simulink model "OMPC"  (R2022b)
settings: Solver=ode5  StartTime=0.0  StopTime=50  FixedStep=Ts  RelTol=1e-3
values from neighbouring files (symbols this model uses):
  A = [A zeros(nA, nAm); zeros(nAm, nA) Am]    [generateFloor.m]    (also in model_floorConjuction.m = A0; model_levelConjuction.m = A0; ompc_data.m = [-0.9146 0 0.0405)
  B = [B zeros(nA, nBm); zeros(nAm, nB) Bm]    [generateFloor.m]    (also in model_floorConjuction.m = B0; model_levelConjuction.m = B0; ompc_data.m = [0.0544 -0.0757)
  Bd = Bd(:, 1:size(B, 2))    [plik_generujDane.m]
  C = [C zeros(nC, nAm); zeros(nCm, nA) Cm]    [generateFloor.m]    (also in model_floorConjuction.m = C0; model_levelConjuction.m = C0; ompc_data.m = [0.3 0.01 -0.05)
  D = Dm    [generateFloor.m]    (also in ompc_data.m = zeros(size(C,1),size(B,2)))
  G = G'    [ompc_data.m]
  nc = 4    [ompc_data.m]    (also in plik_generujDane.m = 60)
  npred = 20    [ompc_data.m]    (also in plik_generujDane.m = 120)
  nu = size(B,2)    [ompc_cost.m]    (also in ompc_cost_tracking.m; ompc_data.m; ompc_law.m; ompc_law_tracking.m)
  nx = size(B,1)    [ompc_cost.m]    (also in ompc_cost_tracking.m = size(A,1); ompc_data.m = size(A,1); ompc_law.m = size(A,1); ompc_law_tracking.m = size(A,1))
  Sc = Spsi(nx+1:end,nx+1:end)    [ompc_cost.m]    (also in ompc_cost_tracking.m = Spsi(nx+1:nx+nuc,nx+1:nx+nuc); ompc_law.m = (Sc+Sc')/2; ompc_law_tracking.m = (Sc+Sc')/2)
  Sx = Spsi(1:nx,1:nx)    [ompc_cost.m]    (also in ompc_cost_tracking.m)
  Sxc = Spsi(1:nx,nx+1:end)    [ompc_cost.m]    (also in ompc_cost_tracking.m = Spsi(1:nx,nx+1:nx+nuc))
  Ts = 0.1    [ompc_data.m]    (also in plik_generujDane.m = 720)
  umax = 13*ones(size(Bd,2),1)    [ompc_data.m]    (also in plik_generujDane.m = 45*ones(nu,1))
  umin = -10*ones(size(Bd,2),1)    [ompc_data.m]    (also in plik_generujDane.m = 19*ones(nu,1))
  xmax = [5;5;5]    [ompc_data.m]    (also in plik_generujDane.m = xmax')
  xmin = [-13.5;-13.5;-13]    [ompc_data.m]    (also in plik_generujDane.m = xmin')
  ymax = 2*ones(size(Cd,1),1)    [ompc_data.m]    (also in plik_generujDane.m = Ta_max*ones(ny,1))
  ymin = -0.1*ones(size(Cd,1),1)    [ompc_data.m]    (also in plik_generujDane.m = Ta_min*ones(ny,1))
undefined symbols (not defined in the file or in its folder): Ad, Cd, K
libraries: eeStairGenerator x3, simulink x1
settings Model: Creator=artur  LastModifiedBy=artur

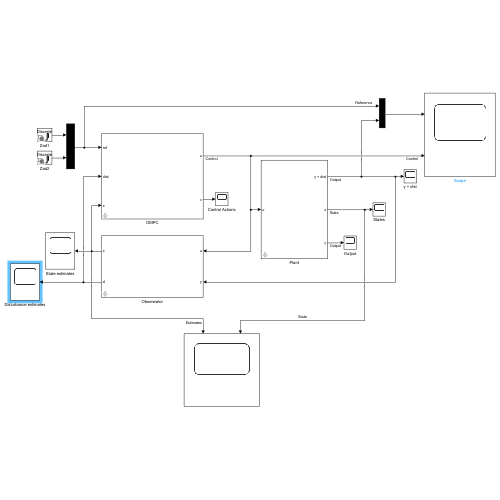
[thumbnail: Simulink's stored preview of the top-level diagram]
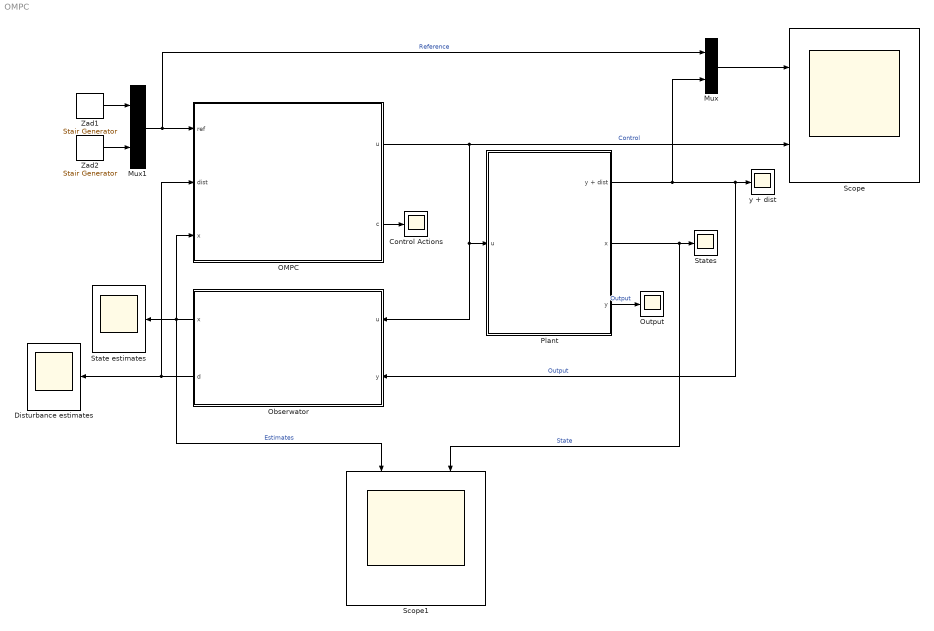
== system OMPC ==
  Control Actions : Scope
  Disturbance estimates : Scope
  Mux : Mux  Inputs=2
  Mux1 : Mux  Inputs=2
  OMPC : Subsystem  mask{A=Ad, B=Bd, C=Cd, nc=nc, npred=npred, Sx=Sx, Sxc=Sxc, Sc=Sc, K=K, umax=umax, umin=umin, ymax=ymax, ymin=ymin, xmax=xmax, xmin=xmin}
      mask prompts: A "Macierz A"; B "Macierz  B"; C "Macierz C"; nc "Liczba zmiennych decyzyjnych"; npred "Horyzont predykcji"; Sx "Macierz Sx"; Sxc "Macierz Sxc"; Sc "Macierz Sc"; K "Macierz K"
      mask DialogControl ParameterGroupVar Prompt: Parametry modelu
      mask DialogControl Container3 Prompt: Parametry regulatora
      mask DialogControl Container4 Prompt: Ograniczenia
  Obserwator : Subsystem  mask{A=Ad, B=Bd, C=Cd, G=G}
      mask prompts: A "Macierz A"; B "Macierz B"; C "Macierz C"; G "Macierz G"
  Output : Scope
  Plant : Subsystem  mask{A=A, B=B, C=C, D=D}
      mask prompts: A "Macierz A:"; B "Macierz B"; C "Macierz C"; D "Macierz D"
      mask DialogControl ParameterGroupVar Prompt: Parametry modelu
  Scope : Scope  NumInputPorts=2
  Scope1 : Scope  NumInputPorts=2
  State estimates : Scope
  States : Scope
  Zad1 : eeStairGenerator/Stair Generator  LabelModeActiveChoice=Discrete  TimeInput=[0 10 20 30 40 50]  AmplitudeInput=[0.2 0.2 0.2 0.2 0.5 0.5]  SampleTime=Ts  RepeatPattern=on  OutDataTypeStr=double
      settings: LibrarySourceBlock=ee_sl_lib/General Control/Stair Generator
  Zad2 : eeStairGenerator/Stair Generator  LabelModeActiveChoice=Discrete  TimeInput=[0 5 10 15 20 25 30 35 40 45]  AmplitudeInput=[0.1 0.1 0.1 0.1 1 1 1 0.5 0.2 0.2]  SampleTime=Ts  RepeatPattern=on  OutDataTypeStr=double
      settings: LibrarySourceBlock=ee_sl_lib/General Control/Stair Generator
  y + dist : Scope
  wires:
  Plant/2(x) -> States/1, Scope1/2  "State"
  OMPC/1(u) -> Obserwator/1(u), Plant/1(u), Scope/2  "Control"
  Plant/1(y + dist) -> y + dist/1, Obserwator/2(y), Mux/2  "Output"
  Mux1/1 -> Mux/1, OMPC/1(ref)  "Reference"
  Mux/1 -> Scope/1
  OMPC/2(c) -> Control Actions/1
  Obserwator/1(x) -> Scope1/1, State estimates/1, OMPC/3(x)  "Estimates"
  Zad1/1 -> Mux1/1
  Zad2/1 -> Mux1/2
  Obserwator/2(d) -> Disturbance estimates/1, OMPC/2(dist)
  Plant/3(y) -> Output/1  "Output"

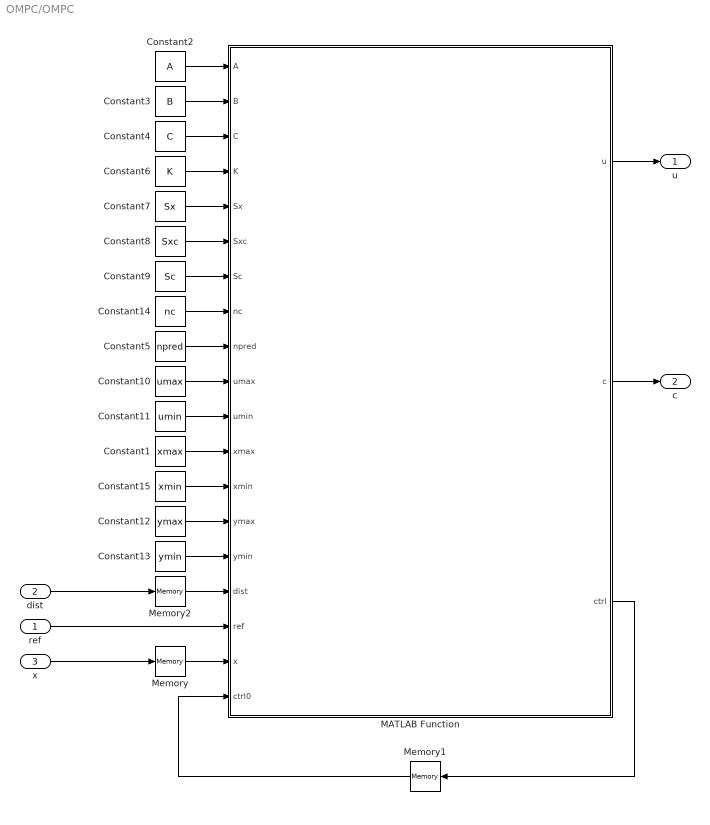
== system OMPC/OMPC ==
  ref : Inport
  dist : Inport  Port=2
  x : Inport  Port=3
  Constant1 : Constant  Value=xmax
  Constant10 : Constant  Value=umax
  Constant11 : Constant  Value=umin
  Constant12 : Constant  Value=ymax
  Constant13 : Constant  Value=ymin
  Constant14 : Constant  Value=nc
  Constant15 : Constant  Value=xmin
  Constant2 : Constant  Value=A
  Constant3 : Constant  Value=B
  Constant4 : Constant  Value=C
  Constant5 : Constant  Value=npred
  Constant6 : Constant  Value=K
  Constant7 : Constant  Value=Sx
  Constant8 : Constant  Value=Sxc
  Constant9 : Constant  Value=Sc
  MATLAB Function : MATLAB Function  TreatAsAtomicUnit=on
  Memory : Memory  InitialCondition=size(nx,1)
  Memory1 : Memory  InitialCondition=zeros(nc*size(B,2),1)
  Memory2 : Memory  InitialCondition=size(nu,1)
  u : Outport
  c : Outport  Port=2
  wires:
  Constant6/1 -> MATLAB Function/4(K)
  Constant9/1 -> MATLAB Function/7(Sc)
  Constant8/1 -> MATLAB Function/6(Sxc)
  Constant2/1 -> MATLAB Function/1(A)
  Constant7/1 -> MATLAB Function/5(Sx)
  Constant4/1 -> MATLAB Function/3(C)
  x/1 -> Memory/1
  Constant3/1 -> MATLAB Function/2(B)
  MATLAB Function/1(u) -> u/1
  ref/1 -> MATLAB Function/17(ref)
  Constant10/1 -> MATLAB Function/10(umax)
  Constant11/1 -> MATLAB Function/11(umin)
  Constant12/1 -> MATLAB Function/14(ymax)
  Constant13/1 -> MATLAB Function/15(ymin)
  Memory/1 -> MATLAB Function/18(x)
  dist/1 -> Memory2/1
  Memory1/1 -> MATLAB Function/19(ctrl0)
  MATLAB Function/3(ctrl) -> Memory1/1
  MATLAB Function/2(c) -> c/1
  Constant5/1 -> MATLAB Function/9(npred)
  Constant14/1 -> MATLAB Function/8(nc)
  Memory2/1 -> MATLAB Function/16(dist)
  Constant15/1 -> MATLAB Function/13(xmin)
  Constant1/1 -> MATLAB Function/12(xmax)

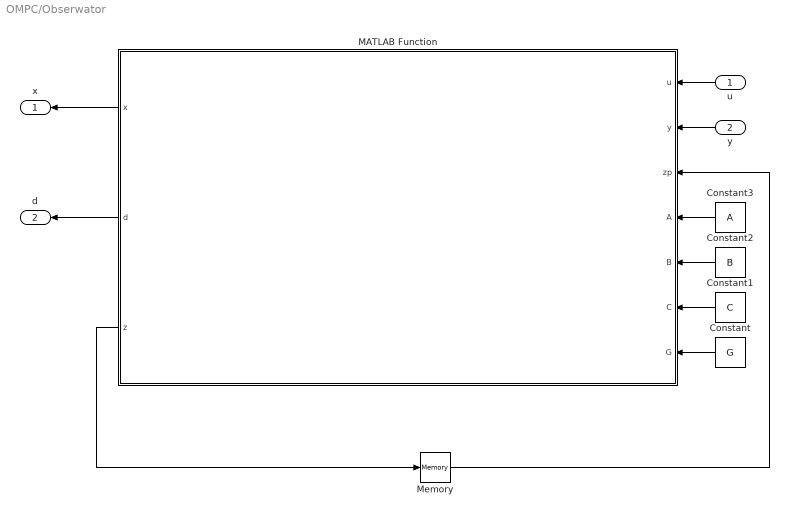
== system OMPC/Obserwator ==
  u : Inport
  y : Inport  Port=2
  Constant : Constant  Value=G
  Constant1 : Constant  Value=C
  Constant2 : Constant  Value=B
  Constant3 : Constant  Value=A
  MATLAB Function : MATLAB Function  TreatAsAtomicUnit=on
  Memory : Memory  InitialCondition=zeros(size(A,1)+size(B,2),1)
  x : Outport
  d : Outport  Port=2
  wires:
  Constant3/1 -> MATLAB Function/4(A)
  Constant1/1 -> MATLAB Function/6(C)
  Constant2/1 -> MATLAB Function/5(B)
  Constant/1 -> MATLAB Function/7(G)
  Memory/1 -> MATLAB Function/3(zp)
  y/1 -> MATLAB Function/2(y)
  u/1 -> MATLAB Function/1(u)
  MATLAB Function/3(z) -> Memory/1
  MATLAB Function/1(x) -> x/1
  MATLAB Function/2(d) -> d/1

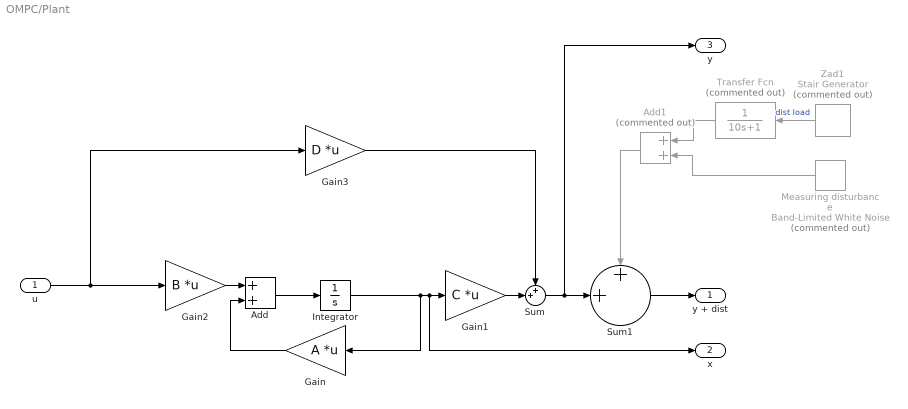
== system OMPC/Plant ==
  u : Inport
  Add : Sum
  Add1 : Sum  Commented=on
  Gain : Gain  Gain=A  Multiplication=Matrix(K*u) (u vector)
  Gain1 : Gain  Gain=C  Multiplication=Matrix(K*u) (u vector)
  Gain2 : Gain  Gain=B  Multiplication=Matrix(K*u) (u vector)
  Gain3 : Gain  Gain=D  Multiplication=Matrix(K*u) (u vector)
  Integrator : Integrator
  Measuring disturbance : simulink/Sources/Band-Limited White Noise  Commented=on  Cov=[0.00002]  Ts=0.1  seed=[23341]
  Sum : Sum  Inputs=++|
  Sum1 : Sum  Inputs=++|
  Transfer Fcn : TransferFcn  Commented=on  Denominator=[10 1]
  Zad1 : eeStairGenerator/Stair Generator  Commented=on  LabelModeActiveChoice=Discrete  TimeInput=[0 5 10 15 20 25 30 35 40 45]  AmplitudeInput=[0 0 0 0 0.1 0.1 0.1 0 0 0]  SampleTime=0.1  RepeatPattern=on  OutDataTypeStr=double
      settings: LibrarySourceBlock=ee_sl_lib/General Control/Stair Generator
  y + dist : Outport
  x : Outport  Port=2
  y : Outport  Port=3
  wires:
  u/1 -> Gain3/1, Gain2/1
  Integrator/1 -> Gain/1, x/1, Gain1/1
  Gain/1 -> Add/2
  Add/1 -> Integrator/1
  Gain2/1 -> Add/1
  Gain1/1 -> Sum/2
  Gain3/1 -> Sum/1
  Sum1/1 -> y + dist/1
  Sum/1 -> y/1, Sum1/2
  Zad1/1 -> Transfer Fcn/1  "dist load"
  Add1/1 -> Sum1/1
  Transfer Fcn/1 -> Add1/1
  Measuring disturbance/1 -> Add1/2

== matlab function OMPC/Obserwator/MATLAB Function ==
  data: u input; x output; y input; zp input; A input; B input; C input; G input; d output; z output
function [x,d,z] = fcn(u,y,zp,A,B,C,G)

nx = size(A,1);
nu = size(B,2);
ny = size(C,1);

Ao = [A zeros(nx,nu);zeros(nu,nx) eye(nu)];
Bo = [B;zeros(nu)];
Co = [C eye(nu)];
Go = [G;[0.01 0.02;0.035 0.2]];


z = (Ao - Go*Co)*zp + [Bo,Go]*[u;y];

x = z(1:nx,:);
d = z(nx+1:end,:);

== matlab function OMPC/MATLAB Function ==
  data: A input; B input; C input; K input; Sx input; Sxc input; Sc input; nc input; npred input; umax input; umin input; xmax input; xmin input; ymax input; ymin input; dist input; ref input; x input; ctrl0 input; u output; c output; ctrl output
function [u,c,ctrl] = fcn(A,B,C,K,Sx,Sxc,Sc,nc,npred,umax,umin,xmax,xmin,ymax,ymin,dist,ref,x,ctrl0)

% [u,c] = ompc_law_unconstrained(A,B,C,K,Sx,Sxc,Sc,ref,dist,x);

[u,ctrl] = ompc_law(A,B,C,K,Sx,Sxc,Sc,umax,umin,xmax,xmin,ymax,ymin,nc,npred,ref,dist,ctrl0,x);
c = ctrl(1:size(B,2),:);
